simulink model "PowerController"  (R2024b)
settings: configuration reference "STM32H7_Config" (kept outside this file)
undefined symbols (not defined in the file): MNominal, NKe, NPowerControllerIntegralGain, PPowerControllerIntegralLowerLimit, PPowerControllerIntegralTermActivation, PPowerControllerIntegralUpperLimit, PPowerControllerProportionalLowerLimit, PPowerControllerProportionalUpperLimit, tTorqueControlTask
libraries: simulink x6
settings Model: DataDictionary=Master_Dictionary.sldd  EnableAccessToBaseWorkspace=off  Creator=torni  LastModifiedBy=William
settings ConfigSetRef: SourceName=STM32H7_Config

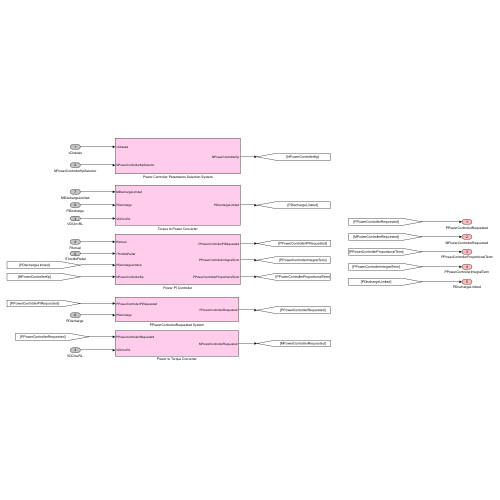
[thumbnail: Simulink's stored preview of the top-level diagram]
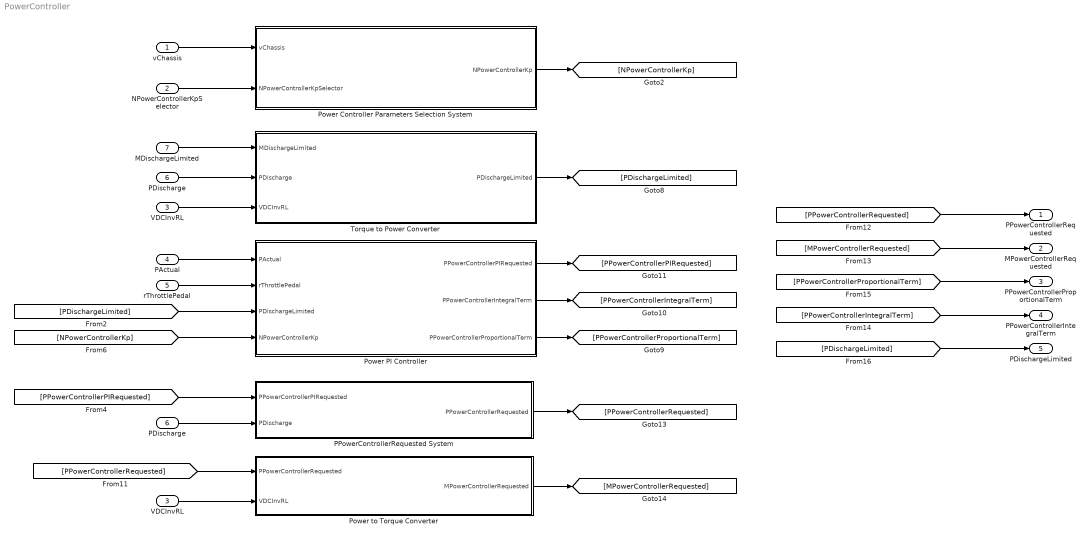
== system PowerController ==
  vChassis : Inport  OutDataTypeStr=double
  NPowerControllerKpSelector : Inport  Port=2  OutDataTypeStr=double
  VDCInvRL : Inport  Port=3  OutDataTypeStr=double
  PActual : Inport  Port=4  OutDataTypeStr=double
  rThrottlePedal : Inport  Port=5  OutDataTypeStr=double
  PDischarge : Inport  Port=6  OutDataTypeStr=double
  MDischargeLimited : Inport  Port=7  OutDataTypeStr=double
  "PDischarge " : InportShadow  Port=6  OutDataTypeStr=double
  PPowerControllerRequested System : Subsystem
  Power Controller Parameters Selection System : Subsystem
  Power PI Controller : Subsystem
  Power to Torque Converter : Subsystem
  Torque to Power Converter : Subsystem
  "VDCInvRL " : InportShadow  Port=3  OutDataTypeStr=double
  PPowerControllerRequested : Outport  OutDataTypeStr=double  VectorParamsAs1DForOutWhenUnconnected=off
  MPowerControllerRequested : Outport  Port=2  OutDataTypeStr=double  VectorParamsAs1DForOutWhenUnconnected=off
  PPowerControllerProportionalTerm : Outport  Port=3  OutDataTypeStr=double  VectorParamsAs1DForOutWhenUnconnected=off
  PPowerControllerIntegralTerm : Outport  Port=4  OutDataTypeStr=double  VectorParamsAs1DForOutWhenUnconnected=off
  PDischargeLimited : Outport  Port=5  OutDataTypeStr=double  VectorParamsAs1DForOutWhenUnconnected=off
  wires:
  VDCInvRL/1 -> Torque to Power Converter/3(VDCInvRL)
  vChassis/1 -> Power Controller Parameters Selection System/1(vChassis)
  "VDCInvRL "/1 -> Power to Torque Converter/2(VDCInvRL)
  PDischarge/1 -> Torque to Power Converter/2(PDischarge)
  Power Controller Parameters Selection System/1(NPowerControllerKp) -> [NPowerControllerKp]
  MDischargeLimited/1 -> Torque to Power Converter/1(MDischargeLimited)
  Torque to Power Converter/1(PDischargeLimited) -> [PDischargeLimited]
  NPowerControllerKpSelector/1 -> Power Controller Parameters Selection System/2(NPowerControllerKpSelector)
  PActual/1 -> Power PI Controller/1(PActual)
  rThrottlePedal/1 -> Power PI Controller/2(rThrottlePedal)
  [PDischargeLimited] -> PDischargeLimited/1
  [PPowerControllerProportionalTerm] -> PPowerControllerProportionalTerm/1
  [PPowerControllerIntegralTerm] -> PPowerControllerIntegralTerm/1
  [PDischargeLimited] -> Power PI Controller/3(PDischargeLimited)
  Power PI Controller/3(PPowerControllerProportionalTerm) -> [PPowerControllerProportionalTerm]
  Power PI Controller/2(PPowerControllerIntegralTerm) -> [PPowerControllerIntegralTerm]
  Power PI Controller/1(PPowerControllerPIRequested) -> [PPowerControllerPIRequested]
  [NPowerControllerKp] -> Power PI Controller/4(NPowerControllerKp)
  [PPowerControllerPIRequested] -> PPowerControllerRequested System/1(PPowerControllerPIRequested)
  PPowerControllerRequested System/1(PPowerControllerRequested) -> [PPowerControllerRequested]
  [PPowerControllerRequested] -> Power to Torque Converter/1(PPowerControllerRequested)
  Power to Torque Converter/1(MPowerControllerRequested) -> [MPowerControllerRequested]
  [PPowerControllerRequested] -> PPowerControllerRequested/1
  [MPowerControllerRequested] -> MPowerControllerRequested/1
  "PDischarge "/1 -> PPowerControllerRequested System/2(PDischarge)

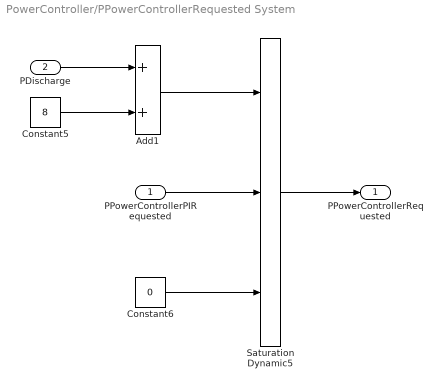
== system PowerController/PPowerControllerRequested System ==
  PPowerControllerPIRequested : Inport  OutDataTypeStr=double
  PDischarge : Inport  Port=2  OutDataTypeStr=double
  Add1 : Sum
  Constant5 : Constant  Value=8
  Constant6 : Constant  Value=0  SampleTime=-1
  Saturation Dynamic5 : simulink/Discontinuities/Saturation Dynamic  OutMin=[]  OutMax=[]  OutDataTypeStr=Inherit: Same as second input  OutDataType=fixdt(1, 16)  OutScaling=2^-10  DoSatur=off
  PPowerControllerRequested : Outport  OutDataTypeStr=double  VectorParamsAs1DForOutWhenUnconnected=off
  wires:
  Constant6/1 -> Saturation Dynamic5/3
  PPowerControllerPIRequested/1 -> Saturation Dynamic5/2
  Add1/1 -> Saturation Dynamic5/1
  Saturation Dynamic5/1 -> PPowerControllerRequested/1
  Constant5/1 -> Add1/2
  PDischarge/1 -> Add1/1

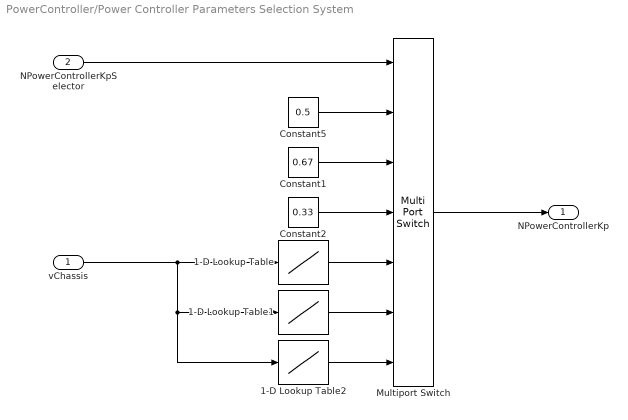
== system PowerController/Power Controller Parameters Selection System ==
  vChassis : Inport  OutDataTypeStr=double
  NPowerControllerKpSelector : Inport  Port=2  OutDataTypeStr=double
  1-D Lookup Table : Lookup_n-D  NumberOfTableDimensions=1  BreakpointsForDimension1=[0,23.9,24,40]  Table=[0.5,0.5,0.1,0.1]  InternalRulePriority=Speed  RndMeth=Simplest
  1-D Lookup Table1 : Lookup_n-D  NumberOfTableDimensions=1  BreakpointsForDimension1=[0,23.9,24,40]  Table=[0.67,0.67,0.13,0.13]  InternalRulePriority=Speed  RndMeth=Simplest
  1-D Lookup Table2 : Lookup_n-D  NumberOfTableDimensions=1  BreakpointsForDimension1=[0,23.9,24,40]  Table=[0.5,0.5,0.01,0.01]  InternalRulePriority=Speed  RndMeth=Simplest
  Constant1 : Constant  Value=0.67
  Constant2 : Constant  Value=0.33
  Constant5 : Constant  Value=0.5
  Multiport Switch : MultiPortSwitch  Inputs=6  SaturateOnIntegerOverflow=off  InputSameDT=off
  NPowerControllerKp : Outport  OutDataTypeStr=double  VectorParamsAs1DForOutWhenUnconnected=off
  wires:
  Multiport Switch/1 -> NPowerControllerKp/1
  NPowerControllerKpSelector/1 -> Multiport Switch/1
  1-D Lookup Table2/1 -> Multiport Switch/7
  Constant1/1 -> Multiport Switch/3
  Constant2/1 -> Multiport Switch/4
  1-D Lookup Table/1 -> Multiport Switch/5
  1-D Lookup Table1/1 -> Multiport Switch/6
  Constant5/1 -> Multiport Switch/2
  vChassis/1 -> 1-D Lookup Table2/1, 1-D Lookup Table1/1, 1-D Lookup Table/1

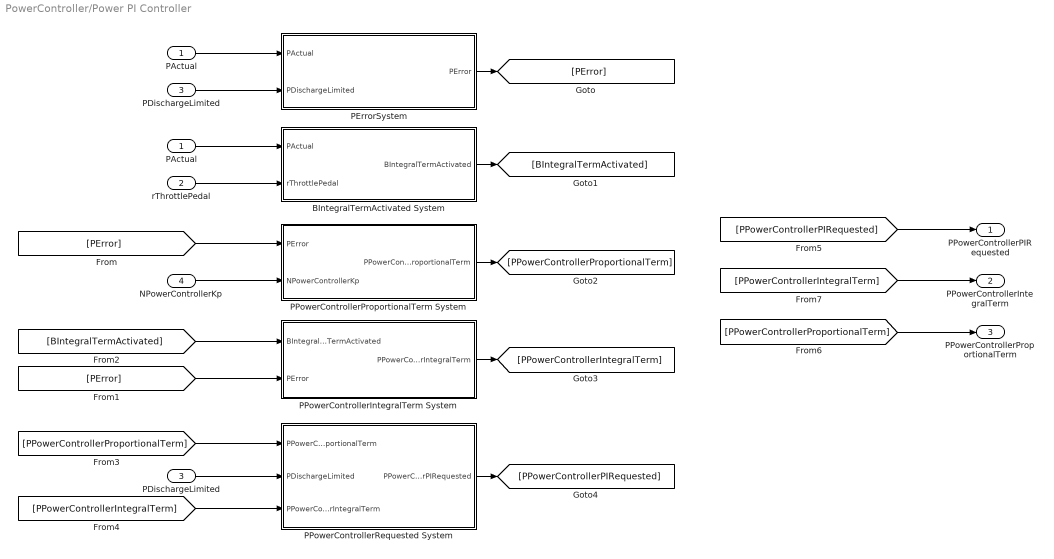
== system PowerController/Power PI Controller ==
  PActual : Inport  OutDataTypeStr=double
  rThrottlePedal : Inport  Port=2  OutDataTypeStr=double
  PDischargeLimited : Inport  Port=3  OutDataTypeStr=double
  NPowerControllerKp : Inport  Port=4  OutDataTypeStr=double
  BIntegralTermActivated System : Subsystem
  "PActual " : InportShadow  OutDataTypeStr=double
  "PDischargeLimited " : InportShadow  Port=3  OutDataTypeStr=double
  PErrorSystem : Subsystem
  PPowerControllerIntegralTerm System : Subsystem
  PPowerControllerProportionalTerm System : Subsystem
  PPowerControllerRequested System : Subsystem
  PPowerControllerPIRequested : Outport  OutDataTypeStr=double  VectorParamsAs1DForOutWhenUnconnected=off
  PPowerControllerIntegralTerm : Outport  Port=2  OutDataTypeStr=double  VectorParamsAs1DForOutWhenUnconnected=off
  PPowerControllerProportionalTerm : Outport  Port=3  OutDataTypeStr=double  VectorParamsAs1DForOutWhenUnconnected=off
  wires:
  PActual/1 -> BIntegralTermActivated System/1(PActual)
  rThrottlePedal/1 -> BIntegralTermActivated System/2(rThrottlePedal)
  "PActual "/1 -> PErrorSystem/1(PActual)
  PDischargeLimited/1 -> PErrorSystem/2(PDischargeLimited)
  PPowerControllerProportionalTerm System/1(PPowerControllerProportionalTerm) -> [PPowerControllerProportionalTerm]
  PErrorSystem/1(PError) -> [PError]
  [PError] -> PPowerControllerProportionalTerm System/1(PError)
  BIntegralTermActivated System/1(BIntegralTermActivated) -> [BIntegralTermActivated]
  PPowerControllerIntegralTerm System/1(PPowerControllerIntegralTerm) -> [PPowerControllerIntegralTerm]
  NPowerControllerKp/1 -> PPowerControllerProportionalTerm System/2(NPowerControllerKp)
  [PError] -> PPowerControllerIntegralTerm System/2(PError)
  [BIntegralTermActivated] -> PPowerControllerIntegralTerm System/1(BIntegralTermActivated)
  "PDischargeLimited "/1 -> PPowerControllerRequested System/2(PDischargeLimited)
  [PPowerControllerProportionalTerm] -> PPowerControllerRequested System/1(PPowerControllerProportionalTerm)
  [PPowerControllerIntegralTerm] -> PPowerControllerRequested System/3(PPowerControllerIntegralTerm)
  PPowerControllerRequested System/1(PPowerControllerPIRequested) -> [PPowerControllerPIRequested]
  [PPowerControllerPIRequested] -> PPowerControllerPIRequested/1
  [PPowerControllerProportionalTerm] -> PPowerControllerProportionalTerm/1
  [PPowerControllerIntegralTerm] -> PPowerControllerIntegralTerm/1

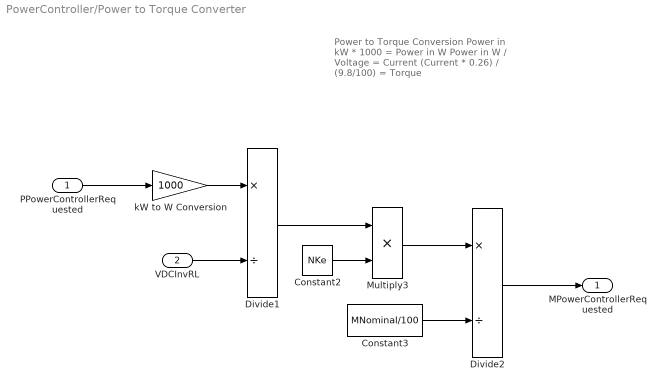
== system PowerController/Power to Torque Converter ==
  note: Power to Torque Conversion
      |
      | Power in kW * 1000 = Power in W
      |
      | Power in W / Voltage = Current
      |
      | (Current * 0.26) / (9.8/100) = Torque
  PPowerControllerRequested : Inport  OutDataTypeStr=double
  VDCInvRL : Inport  Port=2  OutDataTypeStr=double
  Constant2 : Constant  Value=NKe
  Constant3 : Constant  Value=MNominal/100
  Divide1 : Product  Inputs=*/
  Divide2 : Product  Inputs=*/
  Multiply3 : Product
  kW to W Conversion : Gain  Gain=1000
  MPowerControllerRequested : Outport  OutDataTypeStr=double  VectorParamsAs1DForOutWhenUnconnected=off
  wires:
  VDCInvRL/1 -> Divide1/2
  kW to W Conversion/1 -> Divide1/1
  Multiply3/1 -> Divide2/1
  PPowerControllerRequested/1 -> kW to W Conversion/1
  Constant2/1 -> Multiply3/2
  Divide2/1 -> MPowerControllerRequested/1
  Divide1/1 -> Multiply3/1
  Constant3/1 -> Divide2/2

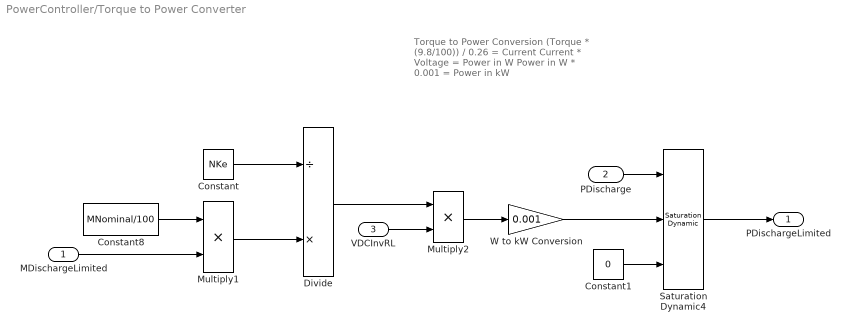
== system PowerController/Torque to Power Converter ==
  note: Torque to Power Conversion
      |
      | (Torque * (9.8/100)) / 0.26 = Current
      |
      | Current * Voltage = Power in W
      |
      | Power in W * 0.001 = Power in kW
  MDischargeLimited : Inport  OutDataTypeStr=double
  PDischarge : Inport  Port=2  OutDataTypeStr=double
  VDCInvRL : Inport  Port=3  OutDataTypeStr=double
  Constant : Constant  Value=NKe
  Constant1 : Constant  Value=0
  Constant8 : Constant  Value=MNominal/100
  Divide : Product  Inputs=/*
  Multiply1 : Product
  Multiply2 : Product
  Saturation Dynamic4 : simulink/Discontinuities/Saturation Dynamic  OutMin=[]  OutMax=[]  OutDataTypeStr=double  OutputDataTypeScalingMode=double  OutDataType=fixdt(1, 16)  OutScaling=2^-10  DoSatur=off
  W to kW Conversion : Gain  Gain=0.001
  PDischargeLimited : Outport  OutDataTypeStr=double  VectorParamsAs1DForOutWhenUnconnected=off
  wires:
  Divide/1 -> Multiply2/1
  Constant8/1 -> Multiply1/1
  MDischargeLimited/1 -> Multiply1/2
  Multiply1/1 -> Divide/2
  PDischarge/1 -> Saturation Dynamic4/1
  Multiply2/1 -> W to kW Conversion/1
  VDCInvRL/1 -> Multiply2/2
  Constant1/1 -> Saturation Dynamic4/3
  Saturation Dynamic4/1 -> PDischargeLimited/1
  Constant/1 -> Divide/1
  W to kW Conversion/1 -> Saturation Dynamic4/2

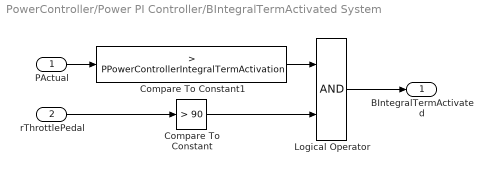
== system PowerController/Power PI Controller/BIntegralTermActivated System ==
  PActual : Inport  OutDataTypeStr=double
  rThrottlePedal : Inport  Port=2  OutDataTypeStr=double
  Compare To Constant : simulink/Logic and Bit Operations/Compare To Constant  relop=>  const=90  OutDataTypeStr=boolean
  Compare To Constant1 : simulink/Logic and Bit Operations/Compare To Constant  relop=>  const=PPowerControllerIntegralTermActivation  OutDataTypeStr=boolean
  Logical Operator : Logic  AllPortsSameDT=off  OutDataTypeStr=boolean
  BIntegralTermActivated : Outport  OutDataTypeStr=boolean  VectorParamsAs1DForOutWhenUnconnected=off
  wires:
  rThrottlePedal/1 -> Compare To Constant/1
  PActual/1 -> Compare To Constant1/1
  Compare To Constant1/1 -> Logical Operator/1
  Compare To Constant/1 -> Logical Operator/2
  Logical Operator/1 -> BIntegralTermActivated/1

== system PowerController/Power PI Controller/PErrorSystem ==
  PActual : Inport  OutDataTypeStr=double
  PDischargeLimited : Inport  Port=2  OutDataTypeStr=double
  Subtract : Sum  Inputs=+-
  PError : Outport  OutDataTypeStr=double  VectorParamsAs1DForOutWhenUnconnected=off
  wires:
  PActual/1 -> Subtract/2
  PDischargeLimited/1 -> Subtract/1
  Subtract/1 -> PError/1

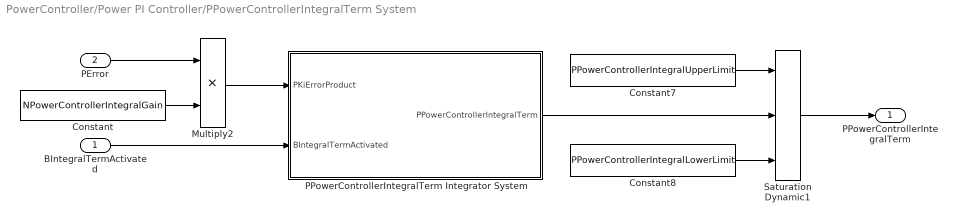
== system PowerController/Power PI Controller/PPowerControllerIntegralTerm System ==
  BIntegralTermActivated : Inport  OutDataTypeStr=boolean
  PError : Inport  Port=2  OutDataTypeStr=double
  Constant : Constant  Value=NPowerControllerIntegralGain
  Constant7 : Constant  Value=PPowerControllerIntegralUpperLimit
  Constant8 : Constant  Value=PPowerControllerIntegralLowerLimit
  Multiply2 : Product
  PPowerControllerIntegralTerm Integrator System : Subsystem
  Saturation Dynamic1 : simulink/Discontinuities/Saturation Dynamic  OutMin=[]  OutMax=[]  OutDataTypeStr=Inherit: Same as second input  OutDataType=fixdt(1, 16)  OutScaling=2^-10  DoSatur=off
  PPowerControllerIntegralTerm : Outport  OutDataTypeStr=double  VectorParamsAs1DForOutWhenUnconnected=off
  wires:
  BIntegralTermActivated/1 -> PPowerControllerIntegralTerm Integrator System/2(BIntegralTermActivated)
  Constant/1 -> Multiply2/2
  Multiply2/1 -> PPowerControllerIntegralTerm Integrator System/1(PKiErrorProduct)
  PError/1 -> Multiply2/1
  Saturation Dynamic1/1 -> PPowerControllerIntegralTerm/1
  PPowerControllerIntegralTerm Integrator System/1(PPowerControllerIntegralTerm) -> Saturation Dynamic1/2
  Constant7/1 -> Saturation Dynamic1/1
  Constant8/1 -> Saturation Dynamic1/3

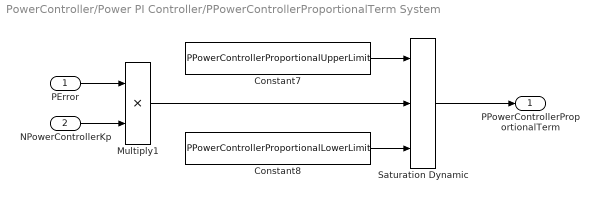
== system PowerController/Power PI Controller/PPowerControllerProportionalTerm System ==
  PError : Inport  OutDataTypeStr=double
  NPowerControllerKp : Inport  Port=2  OutDataTypeStr=double
  Constant7 : Constant  Value=PPowerControllerProportionalUpperLimit
  Constant8 : Constant  Value=PPowerControllerProportionalLowerLimit
  Multiply1 : Product
  Saturation Dynamic : simulink/Discontinuities/Saturation Dynamic  OutMin=[]  OutMax=[]  OutDataTypeStr=Inherit: Same as second input  OutDataType=fixdt(1, 16)  OutScaling=2^-10  DoSatur=off
  PPowerControllerProportionalTerm : Outport  OutDataTypeStr=double  VectorParamsAs1DForOutWhenUnconnected=off
  wires:
  Constant8/1 -> Saturation Dynamic/3
  NPowerControllerKp/1 -> Multiply1/2
  Saturation Dynamic/1 -> PPowerControllerProportionalTerm/1
  PError/1 -> Multiply1/1
  Multiply1/1 -> Saturation Dynamic/2
  Constant7/1 -> Saturation Dynamic/1

== system PowerController/Power PI Controller/PPowerControllerRequested System ==
  PPowerControllerProportionalTerm : Inport  OutDataTypeStr=double
  PDischargeLimited : Inport  Port=2  OutDataTypeStr=double
  PPowerControllerIntegralTerm : Inport  Port=3  OutDataTypeStr=double
  Add : Sum  Inputs=3
  PPowerControllerPIRequested : Outport  VectorParamsAs1DForOutWhenUnconnected=off
  wires:
  PPowerControllerProportionalTerm/1 -> Add/2
  PPowerControllerIntegralTerm/1 -> Add/3
  Add/1 -> PPowerControllerPIRequested/1
  PDischargeLimited/1 -> Add/1

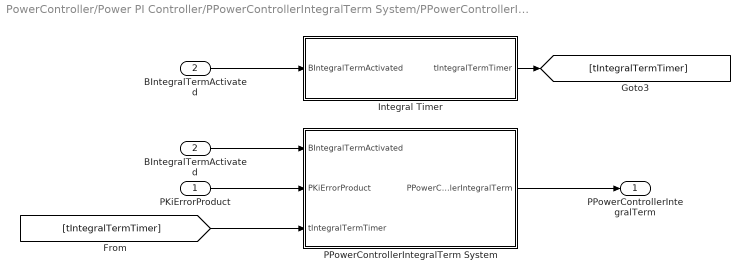
== system PowerController/Power PI Controller/PPowerControllerIntegralTerm System/PPowerControllerIntegralTerm Integrator System ==
  PKiErrorProduct : Inport  OutDataTypeStr=double
  BIntegralTermActivated : Inport  Port=2  OutDataTypeStr=boolean
  "BIntegralTermActivated " : InportShadow  Port=2  OutDataTypeStr=boolean
  Integral Timer : Subsystem
  PPowerControllerIntegralTerm System : Subsystem
  PPowerControllerIntegralTerm : Outport  OutDataTypeStr=double  VectorParamsAs1DForOutWhenUnconnected=off
  wires:
  BIntegralTermActivated/1 -> Integral Timer/1(BIntegralTermActivated)
  "BIntegralTermActivated "/1 -> PPowerControllerIntegralTerm System/1(BIntegralTermActivated)
  PKiErrorProduct/1 -> PPowerControllerIntegralTerm System/2(PKiErrorProduct)
  PPowerControllerIntegralTerm System/1(PPowerControllerIntegralTerm) -> PPowerControllerIntegralTerm/1
  Integral Timer/1(tIntegralTermTimer) -> [tIntegralTermTimer]
  [tIntegralTermTimer] -> PPowerControllerIntegralTerm System/3(tIntegralTermTimer)

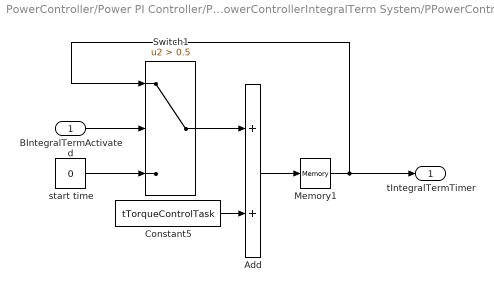
== system PowerController/Power PI Controller/PPowerControllerIntegralTerm System/PPowerControllerIntegralTerm Integrator System/Integral Timer ==
  BIntegralTermActivated : Inport  OutDataTypeStr=boolean
  Add : Sum
  Constant5 : Constant  Value=tTorqueControlTask
  Memory1 : Memory  InheritSampleTime=on
  Switch1 : Switch  Criteria=u2 > Threshold  Threshold=0.5  SaturateOnIntegerOverflow=off  InputSameDT=off
  start time : Constant  Value=0  SampleTime=-1
  tIntegralTermTimer : Outport  OutDataTypeStr=double  VectorParamsAs1DForOutWhenUnconnected=off
  wires:
  Memory1/1 -> Switch1/1, tIntegralTermTimer/1
  BIntegralTermActivated/1 -> Switch1/2
  start time/1 -> Switch1/3
  Switch1/1 -> Add/1
  Constant5/1 -> Add/2
  Add/1 -> Memory1/1

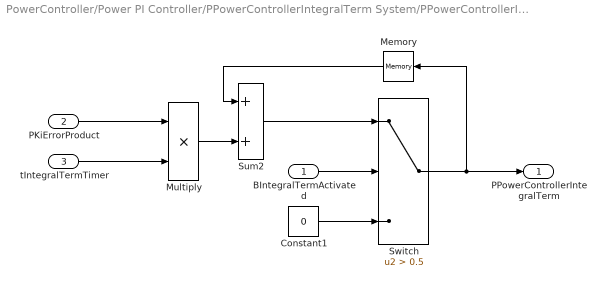
== system PowerController/Power PI Controller/PPowerControllerIntegralTerm System/PPowerControllerIntegralTerm Integrator System/PPowerControllerIntegralTerm System ==
  BIntegralTermActivated : Inport  OutDataTypeStr=boolean
  PKiErrorProduct : Inport  Port=2  OutDataTypeStr=double
  tIntegralTermTimer : Inport  Port=3  OutDataTypeStr=double
  Constant1 : Constant  Value=0
  Memory : Memory  InheritSampleTime=on
  Multiply : Product
  Sum2 : Sum  InputSameDT=on  SaturateOnIntegerOverflow=on  OutDataTypeStr=Inherit: Same as first input
  Switch : Switch  Criteria=u2 > Threshold  Threshold=0.5  SaturateOnIntegerOverflow=off  InputSameDT=off
  PPowerControllerIntegralTerm : Outport  OutDataTypeStr=double  VectorParamsAs1DForOutWhenUnconnected=off
  wires:
  Constant1/1 -> Switch/3
  BIntegralTermActivated/1 -> Switch/2
  tIntegralTermTimer/1 -> Multiply/2
  Multiply/1 -> Sum2/2
  PKiErrorProduct/1 -> Multiply/1
  Switch/1 -> PPowerControllerIntegralTerm/1, Memory/1
  Sum2/1 -> Switch/1
  Memory/1 -> Sum2/1
